simulink model "trigger"  (R2012b)
settings: Solver=ode45  StartTime=0.0  StopTime=inf  RelTol=1e-3
settings Model: Creator=Vicon CS  LastModifiedBy=Vicon CS

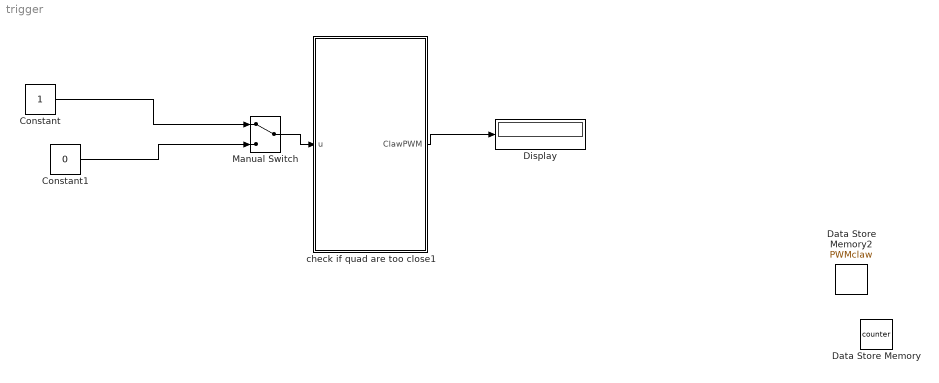
== system trigger ==
  Constant : Constant
  Constant1 : Constant  Value=0
  Data Store Memory : DataStoreMemory  DataStoreName=counter  InitialValue=25  OutDataTypeStr=double
  Data Store Memory2 : DataStoreMemory  DataStoreName=PWMclaw  InitialValue=1690  OutDataTypeStr=double
  Display : Display
  Manual Switch : ManualSwitch
  check if quad are too close1 : MATLAB Function  TreatAsAtomicUnit=on
  wires:
  check if quad are too close1/1(ClawPWM) -> Display/1
  Manual Switch/1 -> check if quad are too close1/1(u)
  Constant/1 -> Manual Switch/1
  Constant1/1 -> Manual Switch/2

== matlab function trigger/check if quad are too close1 ==
  data: u input; ClawPWM output; counter data_store_memory; PWMclaw data_store_memory
function ClawPWM = CLAW(u)
global counter;
global PWMclaw;

if(u~=1)
    if(PWMclaw==1690)
        counter = 1;
        ClawPWM = PWMclaw;       
    elseif (PWMclaw==1200)
        counter = 0;
        ClawPWM = PWMclaw;
    end
    
else
    if(counter==1)
        PWMclaw = 1200;
        ClawPWM = PWMclaw;
    elseif(counter==0)
        PWMclaw = 1690;
        ClawPWM = PWMclaw;
    end
    
end

ClawPWM = PWMclaw;
   
end
